simulink subsystem "subsys_force"  (R2021a)
settings: Solver=VariableStepAuto  StartTime=0.0  StopTime=10.0  RelTol=1e-3
undefined symbols (not defined in the file): be, poly_ae, poly_as
settings Model: Creator=antho  LastModifiedBy=dupa1607

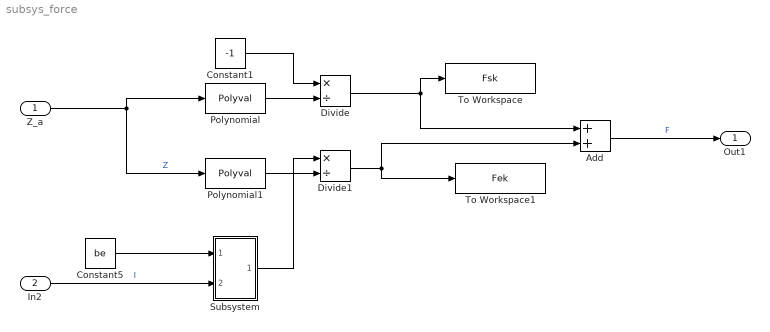
== system subsys_force ==
  Z_a : Inport
  In2 : Inport  Port=2
  Add : Sum
  Constant1 : Constant  Value=-1
  Constant5 : Constant  Value=be
  Divide : Product  Inputs=*/
  Divide1 : Product  Inputs=*/
  Polynomial : Polyval  Coefs=poly_as
  Polynomial1 : Polyval  Coefs=poly_ae
  Subsystem : Subsystem
  To Workspace : ToWorkspace  VariableName=Fsk  SaveFormat=Timeseries  SampleTime=-1
  To Workspace1 : ToWorkspace  VariableName=Fek  SaveFormat=Timeseries  SampleTime=-1
  Out1 : Outport
  wires:
  Divide/1 -> To Workspace/1, Add/1
  Constant5/1 -> Subsystem/1(In1)
  In2/1 -> Subsystem/2(In2)  "I"
  Subsystem/1(Out1) -> Divide1/1
  Z_a/1 -> Polynomial/1, Polynomial1/1  "Z"
  Polynomial1/1 -> Divide1/2
  Constant1/1 -> Divide/1
  Divide1/1 -> Add/2, To Workspace1/1
  Add/1 -> Out1/1  "F"
  Polynomial/1 -> Divide/2

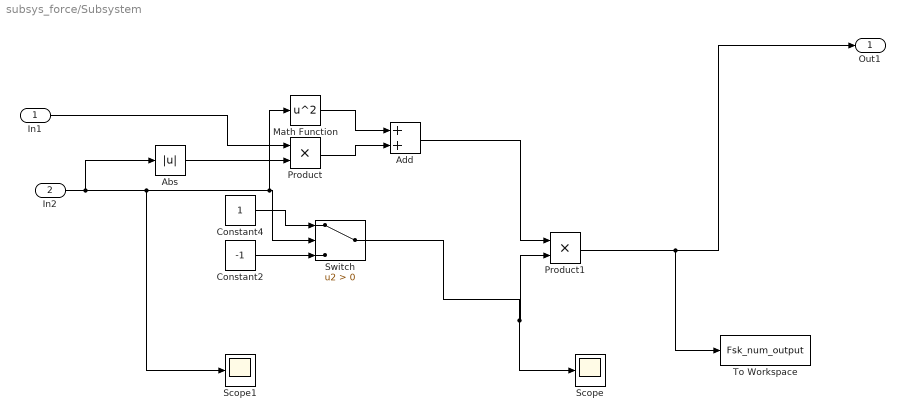
== system subsys_force/Subsystem ==
  In1 : Inport
  In2 : Inport  Port=2
  Abs : Abs
  Add : Sum
  Constant2 : Constant  Value=-1
  Constant4 : Constant
  Math Function : Math  Operator=square  SaturateOnIntegerOverflow=on
  Product : Product
  Product1 : Product
  Scope : Scope
  Scope1 : Scope
  Switch : Switch  Criteria=u2 > Threshold
  To Workspace : ToWorkspace  VariableName=Fsk_num_output  SaveFormat=Timeseries  SampleTime=-1
  Out1 : Outport
  wires:
  Constant4/1 -> Switch/1
  Abs/1 -> Product/2
  Math Function/1 -> Add/1
  Product/1 -> Add/2
  In1/1 -> Product/1
  Add/1 -> Product1/1
  In2/1 -> Abs/1, Scope1/1, Math Function/1, Switch/2
  Constant2/1 -> Switch/3
  Switch/1 -> Scope/1, Product1/2
  Product1/1 -> To Workspace/1, Out1/1
